simulink model "BuckyWagon_01"  (Simulink 7.7)
settings: Solver=FixedStepDiscrete  StartTime=0.0  StopTime=10.0  RelTol=1e-3
PreLoadFcn:
  | try, eval([bdroot '_setup']); catch, eval('model_setup', ''); end
InitFcn:
  | try, eval([bdroot '_setup']); catch, eval('model_setup', ''); end
undefined symbols (not defined in the file or in its folder): ECU565, High, Low, miniviewSetup, motohawk_build_version, motohawk_get_faults, motohawk_setup_toolchains, motohawk_trunc_name, motohawk_vardec_config_group, motohawk_vardec_path, tc, True
libraries: MotoHawk_lib x594, simulink x27, motohawk_control_primitives_lib x19, miniview_lib x10, MotoHawk_VDOGauge_lib x8, motohawk_engine_lib x5, motohawk_annotations_lib x1
(part 8 of 10)

== system BuckyWagon_01/Foreground/Control Strategy/Drive/HillHold Algorithm ==
  Accel : Inport
  Brake : Inport  Port=2
  Motor_Speed : Inport  Port=3
  Chart : Stateflow chart  TreatAsAtomicUnit=on
  HillHold PI Controller1 : Subsystem
  motohawk_calibration1 : MotoHawk_lib/Calibration & Probing Blocks/motohawk_calibration  nam='HillHoldDisengageBrakePct'  val=0.4  storage=Calibration  show_more=on  name_source=Use Parameter  data_type=Inherit from 'Default Value'  read_level=1  write_level=1  ovr_cals=on  view_as=Number  enum_struct={'Disabled', 'Enabled'}  vector_style=Wide Row  use_help_units=off  help=''  units=''  use_header_enum=off  row_header_enum={}  col_header_enum={}  use_min_max=off  min_val=-inf  max_val=inf  use_precision=off  precision=''  gain=1  offset=0  exp=1  use_mototune_group=off  mototune_group=motohawk_vardec_path(gcb)
  motohawk_calibration2 : MotoHawk_lib/Calibration & Probing Blocks/motohawk_calibration  nam='MinBrakeBedPosforHillHold'  val=0.001  storage=Calibration  show_more=on  name_source=Use Parameter  data_type=Inherit from 'Default Value'  read_level=1  write_level=1  ovr_cals=on  view_as=Number  enum_struct={'Disabled', 'Enabled'}  vector_style=Wide Row  use_help_units=off  help=''  units=''  use_header_enum=off  row_header_enum={}  col_header_enum={}  use_min_max=off  min_val=-inf  max_val=inf  use_precision=off  precision=''  gain=1  offset=0  exp=1  use_mototune_group=off  mototune_group=motohawk_vardec_path(gcb)
  motohawk_probe : MotoHawk_lib/Calibration & Probing Blocks/motohawk_probe  nam='Hill_Hold_On'  show_more=off  name_source=Use Parameter  read_level=1  view_as=Number  enum_struct={'Disabled', 'Enabled'}  vector_style=Wide Row  use_help_units=off  help=''  units=''  use_header_enum=off  row_header_enum={}  col_header_enum={}  use_precision=off  precision=''  gain=1  offset=0  exp=1  use_mototune_group=off  mototune_group=motohawk_vardec_path(gcb)
  HillHoldActive : Outport
  HillHoldTq : Outport  Port=2
  wires:
  Accel/1 -> Chart/1(Accel)
  Brake/1 -> Chart/2(Brake)
  Motor_Speed/1 -> Chart/3(RPM), HillHold PI Controller1/2(RPM)
  motohawk_calibration2/1 -> Chart/4(MinBrakeBedPosforHillHold)
  Chart/1(HillHoldOn) -> HillHoldActive/1, HillHold PI Controller1/1(HillHoldEnable), motohawk_probe/1
  motohawk_calibration1/1 -> Chart/5(HillHoldDisengageBrakePct)
  HillHold PI Controller1/1(HillHoldTq) -> HillHoldTq/1

== system BuckyWagon_01/Foreground/Control Strategy/Drive/Normal Driving ==
  note: This currently does nothing... .005 = 1 clock cycle
  Accel : Inport
  Brake : Inport  Port=2
  SOC : Inport  Port=3
  RPM : Inport  Port=4
  RegenDisabled : Inport  Port=5
  Vehicle Speed : Inport  Port=6
  First Order Low Pass (Tunable) : Subsystem  mask(First-Order Low-Pass Filter (Tunable)){nam='Veh_Speed_Regen_Filter', samp_time=-1, group=motohawk_vardec_path(gcb)}
      mask prompts: nam "Name"; samp_time "Sample Time"; group "MotoTune Group String"
      mask help:
      | Discrete first-order low-pass filter, with calibratable time-constant.
      |
      | If 'Sample Time' is -1, then extra code and RAM will be generated to dynamically calculate dt.
      mask Display:
      | patch([0 0 1 1], [0 0.075 0.075 0], [230/255 0/255 0/255])
      | patch([0 0 1 1], [0.025 0.05 0.05 0.025], [150/255 0/255 0/255])
      | patch([0 0 1 1], [0 0.025 0.025 0], [0/255 0/255 0/255])
      | 
      | disp('1st-Order\nLow Pass');
  First Order Low Pass (Tunable)1 : Subsystem  mask(First-Order Low-Pass Filter (Tunable)){nam='FiltConst', samp_time=-1, group=motohawk_vardec_path(gcb)}
      mask prompts: nam "Name"; samp_time "Sample Time"; group "MotoTune Group String"
      mask help:
      | Discrete first-order low-pass filter, with calibratable time-constant.
      |
      | If 'Sample Time' is -1, then extra code and RAM will be generated to dynamically calculate dt.
      mask Display:
      | patch([0 0 1 1], [0 0.075 0.075 0], [230/255 0/255 0/255])
      | patch([0 0 1 1], [0.025 0.05 0.05 0.025], [150/255 0/255 0/255])
      | patch([0 0 1 1], [0 0.025 0.025 0], [0/255 0/255 0/255])
      | 
      | disp('1st-Order\nLow Pass');
  Logic : Logic  Operator=NOT  AllPortsSameDT=off  OutDataTypeStr=boolean
  Product1 : Product  RndMeth=Zero
  Regen : Subsystem  TreatAsAtomicUnit=on
  Relational Operator2 : RelationalOperator  Operator=>  OutDataTypeStr=boolean
  Switch : Switch  Criteria=u2 ~= 0
  motohawk_calibration1 : MotoHawk_lib/Calibration & Probing Blocks/motohawk_calibration  nam='Max_Slect_Tq_drive'  val=800  storage=Calibration  show_more=off  name_source=Use Parameter  data_type=Inherit from 'Default Value'  read_level=1  write_level=1  ovr_cals=on  view_as=Number  enum_struct={'Disabled', 'Enabled'}  vector_style=Wide Row  use_help_units=off  help=''  units=''  use_header_enum=off  row_header_enum={}  col_header_enum={}  use_min_max=off  min_val=-inf  max_val=inf  use_precision=off  precision=''  gain=1  offset=0  exp=1  use_mototune_group=off  mototune_group=motohawk_vardec_path(gcb)
  motohawk_calibration2 : MotoHawk_lib/Calibration & Probing Blocks/motohawk_calibration  nam='Temp_ped_switchOver'  val=0.005  storage=Calibration  show_more=on  name_source=Use Parameter  data_type=Inherit from 'Default Value'  read_level=1  write_level=1  ovr_cals=on  view_as=Number  enum_struct={'Disabled', 'Enabled'}  vector_style=Wide Row  use_help_units=off  help=''  units=''  use_header_enum=off  row_header_enum={}  col_header_enum={}  use_min_max=off  min_val=-inf  max_val=inf  use_precision=on  precision='1.3'  gain=1  offset=0  exp=1  use_mototune_group=off  mototune_group=motohawk_vardec_path(gcb)
  motohawk_table_1d : MotoHawk_lib/Lookup Tables/motohawk_table_1d  SystemSampleTime=-1  nam='AccelPedalMap'  bp_nam=''  breakpoint_data=[0:.01:1]  table_data="[0\t0\t0\t0.015\t0.03\t0.045\t0.06\t0.075\t0.09\t0.105\t0.12\t0.135\t0.15\t0.165\t0.18\t0.195\t0.21\t0.225\t0.24\t0.255\t0.27\t0.285\t0.3\t0.315\t0.33\t0.345\t0.36\t0.375\t0.39\t0.405\t0.42\t0.435\t0.45\t0.465\t0.48\t0.495\t0.51\t0.525\t0.54\t0.555\t0.57\t0.585\t0.6\t0.615\t0.63\t0.645\t0.66\t0.675\t0.69\t0.7\t0.707106781\t0.714142843\t0.721110255\t0.728010989\t0.734846923\t0.741619849\t0.748331477\t0.754983444\t0.761577311\t0.768114575\t0.774596669\t0.781024968\t0.787400787\t0.793725393\t0.8\t0.806225775\t0.81240384\t0.818535277\t0.824621125\t0.830662386\t0.836660027\t0.842614977\t0.848528137\t0.854400375\t0.860232527\t0.866025404\t0.871779789\t0.877496439\t0.883176087\t0.888819442\t0.894427191\t0.9\t0.905538514\t0.911043358\t0.916515139\t0.921954446\t0.92736185\t0.932737905\t0.938083152\t0.943398113\t0.948683298\t0.953939201\t0.959166305\t0.964365076\t0.969535971\t0.974679434\t0.979795897\t0.98488578\t0.989949494\t0.994987437\t1]"  show_more=on  bp_data_type=Inherit from 'Breakpoint Data'  bp_storage=Constant  table_data_type=Inherit from 'Table Data'  storage=NonAdaptive  read_level=1  write_level=1  ovr_cals=on  use_help=off  help=''  bp_units=''  table_units=''  use_min_max=off  bp_min_val=-inf  bp_max_val=inf  min_val=-inf  max_val=inf  use_precision=on  use_breakpoint=off  b_precision=''  b_gain=1  b_offset=0  b_exp=1  use_table=on  t_precision='1.4'  t_gain=1  t_offset=0  t_exp=1  use_links=off  input_name=''  output_name=''  use_mototune_group=off  mototune_group=motohawk_vardec_path(gcb)
  TorqueReq : Outport
  RegenDisable : Outport  Port=2
  wires:
  First Order Low Pass (Tunable)/1(out) -> Regen/4(RPM)
  Brake/1 -> Regen/2(Brake_Pos)
  motohawk_calibration1/1 -> Product1/1
  Accel/1 -> motohawk_table_1d/1, Relational Operator2/1
  Switch/1 -> TorqueReq/1  "Morot_Torque"
  SOC/1 -> Regen/3(SOC)
  RPM/1 -> First Order Low Pass (Tunable)/1(in)
  RegenDisabled/1 -> Regen/5(RegenDisabled)
  Regen/2(RegenDisable) -> RegenDisable/1  "RegenDisable"
  Product1/1 -> Switch/1
  motohawk_calibration2/1 -> Relational Operator2/2
  Vehicle Speed/1 -> Regen/6(Vehicle Speed)
  Relational Operator2/1 -> Switch/2, Logic/1
  Regen/1(RegenTq) -> First Order Low Pass (Tunable)1/1(in)
  Logic/1 -> Regen/1(switch active)
  First Order Low Pass (Tunable)1/1(out) -> Switch/3
  motohawk_table_1d/1 -> Product1/2

== system BuckyWagon_01/Foreground/Control Strategy/HV Controller/Contacter Controller ==
  Battery OK : Inport  OutDataTypeStr=boolean
  Shutdown Command : Inport  Port=2  OutDataTypeStr=boolean
  Contactor Status : Inport  Port=3  OutDataTypeStr=boolean
  Delay falling edge : Subsystem
  Delay rising edge : Subsystem
  Logical Operator2 : Logic  AllPortsSameDT=off  OutDataTypeStr=boolean
  Logical Operator3 : Logic  Operator=NOT  AllPortsSameDT=off  OutDataTypeStr=boolean
  Logical Operator4 : Logic  Inputs=3  AllPortsSameDT=off  OutDataTypeStr=boolean
  Logical Operator5 : Logic  Operator=NOT  AllPortsSameDT=off  OutDataTypeStr=boolean
  Logical Operator6 : Logic  Operator=NOT  AllPortsSameDT=off  OutDataTypeStr=boolean
  Relational Operator : RelationalOperator  OutDataTypeStr=boolean
  Relational Operator1 : RelationalOperator  OutDataTypeStr=boolean
  Time Since Enabled (With Input)1 : motohawk_control_primitives_lib/Time Since Enabled (With Input)1  SystemSampleTime=-1  nam='Contactor_Disable_Timer'  samp_time=-1  init=0  upperlim=3600*24
  Time Since Enabled (With Input)3 : motohawk_control_primitives_lib/Time Since Enabled (With Input)1  SystemSampleTime=-1  nam='Solectria_Enable_timer'  samp_time=-1  init=0  upperlim=3600*24
  motohawk_calibration : MotoHawk_lib/Calibration & Probing Blocks/motohawk_calibration  nam='Contactor_Disable_Delay'  val=0.5  storage=Calibration  show_more=on  name_source=Use Parameter  data_type=Inherit from 'Default Value'  read_level=1  write_level=1  ovr_cals=on  view_as=Number  enum_struct={'Disabled', 'Enabled'}  vector_style=Wide Row  use_help_units=off  help=''  units=''  use_header_enum=off  row_header_enum={}  col_header_enum={}  use_min_max=on  min_val=0  max_val=10  use_precision=on  precision='1.2'  gain=1  offset=0  exp=1  use_mototune_group=on  mototune_group=motohawk_vardec_path(gcb)
  motohawk_calibration1 : MotoHawk_lib/Calibration & Probing Blocks/motohawk_calibration  nam='Load_Enable_Delay'  val=2  storage=Calibration  show_more=on  name_source=Use Parameter  data_type=Inherit from 'Default Value'  read_level=1  write_level=1  ovr_cals=on  view_as=Number  enum_struct={'Disabled', 'Enabled'}  vector_style=Wide Row  use_help_units=off  help=''  units=''  use_header_enum=off  row_header_enum={}  col_header_enum={}  use_min_max=on  min_val=0  max_val=10  use_precision=on  precision='1.2'  gain=1  offset=0  exp=1  use_mototune_group=on  mototune_group=motohawk_vardec_path(gcb)
  motohawk_data_write : MotoHawk_lib/Data Storage Blocks/motohawk_data_write  source=Lookup By Name  structure=Scalar  operation=Write entire data structure at once  sz_vec=-1  sz_row=3  sz_col=2  typ=boolean  nam='MPRD_KeepAlive'  checkNull=off  write_read_only=off  struct_inst_name='Struct1'  struct_name='MyStruct'
  Contactor Enable : Outport  OutDataTypeStr=boolean
  Load Enable : Outport  Port=2  OutDataTypeStr=boolean
  wires:
  Time Since Enabled (With Input)1/1 -> Relational Operator/1
  Logical Operator3/1 -> Logical Operator4/1
  Time Since Enabled (With Input)3/1 -> Relational Operator1/1
  Relational Operator1/1 -> Logical Operator4/2
  Logical Operator5/1 -> Time Since Enabled (With Input)3/1
  Logical Operator4/1 -> Load Enable/1
  motohawk_calibration/1 -> Relational Operator/2
  motohawk_calibration1/1 -> Relational Operator1/2
  Relational Operator/1 -> Logical Operator6/1
  Logical Operator6/1 -> Logical Operator2/2
  Battery OK/1 -> Delay rising edge/1(In)
  Delay falling edge/1(Out) -> motohawk_data_write/1
  Contactor Status/1 -> Logical Operator4/3
  Delay rising edge/1(Out) -> Logical Operator2/1
  Logical Operator2/1 -> Contactor Enable/1, Delay falling edge/1(In)
  Shutdown Command/1 -> Time Since Enabled (With Input)1/1, Logical Operator5/1, Logical Operator3/1

== system BuckyWagon_01/Foreground/MiniViewDisplay/Down Button/Subsystem ==
  Trigger : TriggerPort  TriggerType=function-call
  Read CAN Message : MotoHawk_lib/CAN Blocks/Read CAN Message  nam=['CAN_' num2str(miniview_CAN_channel)]  bus=-2  msg=miniview_button_down  queue=1  slot='miniview_button_down'  valid=off  stale=off  labelwires=on
  Signal Specification : SignalSpecification  OutDataTypeStr=boolean
  Signal Specification1 : SignalSpecification  OutDataTypeStr=uint8
  Out1 : Outport
  Out2 : Outport  Port=2
  wires:
  Signal Specification1/1 -> Out2/1  "down count"
  Signal Specification/1 -> Out1/1  "down asserted"
  Read CAN Message/2 -> Signal Specification1/1  "down count"
  Read CAN Message/1 -> Signal Specification/1  "down asserted"

== system BuckyWagon_01/Foreground/MiniViewDisplay/GetFaultName/Fault Iterator ==
  function : TriggerPort  TriggerType=function-call
  Unit Delay : UnitDelay  SampleTime=-1
  motohawk_fault_iterator : MotoHawk_lib/Fault Management Blocks/motohawk_fault_iterator  criteria=Active Faults  loop=on
  motohawk_fault_name : MotoHawk_lib/Fault Management Blocks/motohawk_fault_name  width=size(char(motohawk_get_faults),2)+1
  Name : Outport
  valid : Outport  Port=2
  wires:
  motohawk_fault_iterator/2 -> Unit Delay/1, motohawk_fault_name/1
  Unit Delay/1 -> motohawk_fault_iterator/1
  motohawk_fault_iterator/1 -> valid/1
  motohawk_fault_name/1 -> Name/1

== system BuckyWagon_01/Foreground/MiniViewDisplay/Menu Button/Subsystem ==
  Trigger : TriggerPort  TriggerType=function-call
  Read CAN Message : MotoHawk_lib/CAN Blocks/Read CAN Message  nam=['CAN_' num2str(miniview_CAN_channel)]  bus=-2  msg=miniview_button_menu  queue=1  slot='miniview_button_menu'  valid=off  stale=off  labelwires=on
  Signal Specification : SignalSpecification  OutDataTypeStr=boolean
  Signal Specification1 : SignalSpecification  OutDataTypeStr=uint8
  Out1 : Outport
  Out2 : Outport  Port=2
  wires:
  Read CAN Message/1 -> Signal Specification/1  "menu asserted"
  Read CAN Message/2 -> Signal Specification1/1  "menu count"
  Signal Specification/1 -> Out1/1  "menu asserted"
  Signal Specification1/1 -> Out2/1  "menu count"

== system BuckyWagon_01/Foreground/MiniViewDisplay/Send String_efficient/Subsystem ==
  string # : Inport
  string : Inport  Port=2
  Trigger : TriggerPort  TriggerType=function-call
  Demux3 : Demux  Outputs=[7 7 3 1]
  Function-Call Generator : simulink/Ports & Subsystems/Function-Call Generator  sample_time=-1  numberOfIterations=1
  Function-Call Subsystem : Subsystem  TreatAsAtomicUnit=on
  Function-Call Subsystem1 : Subsystem  TreatAsAtomicUnit=on
  Send Substring (page 0) : miniview_lib/Send Substring (page 0)  SystemSampleTime=-1  miniview_CAN_channel=miniview_CAN_channel
  Send Substring (page 1) : miniview_lib/Send Substring (page 1)  SystemSampleTime=-1  miniview_CAN_channel=miniview_CAN_channel
  Send Substring (page 2) : miniview_lib/Send Substring (page 2)  SystemSampleTime=-1  miniview_CAN_channel=miniview_CAN_channel
  Terminator : Terminator
  Terminator1 : Terminator
  wires:
  Demux3/3 -> Send Substring (page 2)/2
  Demux3/2 -> Send Substring (page 1)/2, Function-Call Subsystem1/1(In1)
  Demux3/1 -> Send Substring (page 0)/2, Function-Call Subsystem/1(In1)
  string/1 -> Demux3/1  "string"
  string #/1 -> Send Substring (page 1)/1, Send Substring (page 2)/1, Send Substring (page 0)/1  "string #"
  Function-Call Generator/1 -> Send Substring (page 0)/Trigger
  Send Substring (page 0)/1 -> Function-Call Subsystem/Trigger
  Function-Call Subsystem/1(Out) -> Send Substring (page 1)/Trigger
  Send Substring (page 1)/1 -> Function-Call Subsystem1/Trigger
  Function-Call Subsystem1/1(Out) -> Send Substring (page 2)/Trigger
  Demux3/4 -> Terminator/1
  Send Substring (page 2)/1 -> Terminator1/1

== system BuckyWagon_01/Foreground/MiniViewDisplay/Up Button/Subsystem ==
  Trigger : TriggerPort  TriggerType=function-call
  Read CAN Message : MotoHawk_lib/CAN Blocks/Read CAN Message  nam=['CAN_' num2str(miniview_CAN_channel)]  bus=-2  msg=miniview_button_up  queue=1  slot='miniview_button_up'  valid=off  stale=off  labelwires=on
  Signal Specification : SignalSpecification  OutDataTypeStr=boolean
  Signal Specification1 : SignalSpecification  OutDataTypeStr=uint8
  Up Asserted : Outport
  Up Count : Outport  Port=2
  wires:
  Signal Specification1/1 -> Up Count/1  "up count"
  Signal Specification/1 -> Up Asserted/1  "up asserted"
  Read CAN Message/2 -> Signal Specification1/1  "up count"
  Read CAN Message/1 -> Signal Specification/1  "up asserted"

== system BuckyWagon_01/Foreground/Sensors/Brusa Charger/PluggedInDetect ==
  MainsVolt : Inport
  Thres : Inport  Port=2
  Time : Inport  Port=3
  Chart : Stateflow chart  TreatAsAtomicUnit=on
  Relational Operator : RelationalOperator  Operator=>  OutDataTypeStr=boolean
  pluggedIn : Outport
  wires:
  MainsVolt/1 -> Relational Operator/1
  Thres/1 -> Relational Operator/2
  Chart/1(pluggedIn) -> pluggedIn/1
  Relational Operator/1 -> Chart/2(mainsOn)
  Time/1 -> Chart/1(histTime)

== system BuckyWagon_01/Foreground/Sensors/Eaton HV Charger/PluggedInDetect ==
  MainsVolt : Inport
  Thres : Inport  Port=2
  Time : Inport  Port=3
  Chart : Stateflow chart  TreatAsAtomicUnit=on
  Relational Operator : RelationalOperator  Operator=>  OutDataTypeStr=boolean
  pluggedIn : Outport
  wires:
  MainsVolt/1 -> Relational Operator/1
  Thres/1 -> Relational Operator/2
  Chart/1(pluggedIn) -> pluggedIn/1
  Relational Operator/1 -> Chart/2(mainsOn)
  Time/1 -> Chart/1(histTime)

== system BuckyWagon_01/Foreground/Sensors/Linear Sensor Characterization/If Action Subsystem ==
  In : Inport
  Action Port : ActionPort  ActionType=then
  Out : Outport
  wires:
  In/1 -> Out/1

== system BuckyWagon_01/Foreground/Sensors/Linear Sensor Characterization/If Action Subsystem1 ==
  In : Inport
  Action Port : ActionPort  ActionType=elseif
  Out : Outport
  wires:
  In/1 -> Out/1

== system BuckyWagon_01/Foreground/Sensors/Linear Sensor Characterization/If Action Subsystem2 ==
  In : Inport
  Action Port : ActionPort  ActionType=else
  Out : Outport
  wires:
  In/1 -> Out/1

== system BuckyWagon_01/Foreground/Sensors/Linear Sensor Characterization2/If Action Subsystem ==
  In : Inport
  Action Port : ActionPort  ActionType=then
  Out : Outport
  wires:
  In/1 -> Out/1

== system BuckyWagon_01/Foreground/Sensors/Linear Sensor Characterization2/If Action Subsystem1 ==
  In : Inport
  Action Port : ActionPort  ActionType=elseif
  Out : Outport
  wires:
  In/1 -> Out/1

== system BuckyWagon_01/Foreground/Sensors/Linear Sensor Characterization2/If Action Subsystem2 ==
  In : Inport
  Action Port : ActionPort  ActionType=else
  Out : Outport
  wires:
  In/1 -> Out/1

== system BuckyWagon_01/Main Power Relay/Background/Delay/MotoHawk S-R Flip-Flop ==
  note: MotoHawk S-R Flip-Flop
  S : Inport
  R : Inport  Port=2
  Logical Operator : Logic  Operator=OR  OutDataTypeStr=boolean
  Logical Operator1 : Logic  Operator=NOT  OutDataTypeStr=boolean
  Logical Operator2 : Logic  OutDataTypeStr=boolean
  Logical Operator3 : Logic  Operator=NOT  OutDataTypeStr=boolean
  Signal Specification : SignalSpecification  OutDataTypeStr=boolean
  Signal Specification1 : SignalSpecification  OutDataTypeStr=boolean
  Unit Delay : UnitDelay  X0=ic_bool  SampleTime=-1
  Q : Outport
  !Q : Outport  Port=2
  wires:
  Logical Operator3/1 -> !Q/1
  R/1 -> Signal Specification/1
  S/1 -> Signal Specification1/1
  Signal Specification1/1 -> Logical Operator/2
  Signal Specification/1 -> Logical Operator1/1
  Logical Operator2/1 -> Q/1, Unit Delay/1, Logical Operator3/1
  Unit Delay/1 -> Logical Operator/1
  Logical Operator/1 -> Logical Operator2/1
  Logical Operator1/1 -> Logical Operator2/2

== system BuckyWagon_01/Foreground/Actuators/Analog Out/ReverseInd/Enabled Subsystem ==
  Period (Cnt) : Inport
  Enable : EnablePort  StatesWhenEnabling=reset
  Constant : Constant  OutDataTypeStr=int16
  Gain : Gain  Gain=0.5  OutDataTypeStr=Inherit: Same as input
  Relational Operator : RelationalOperator  Operator=<=  OutDataTypeStr=boolean
  Sum : Sum  Inputs=|+-
  Switch : Switch  Criteria=u2 > Threshold
  Unit Delay : UnitDelay  SampleTime=-1
  Out : Outport  InitialOutput=[0]
  wires:
  Relational Operator/1 -> Out/1
  Gain/1 -> Relational Operator/1
  Period (Cnt)/1 -> Gain/1, Switch/3
  Switch/1 -> Sum/1
  Sum/1 -> Relational Operator/2, Unit Delay/1
  Unit Delay/1 -> Switch/1, Switch/2
  Constant/1 -> Sum/2

== system BuckyWagon_01/Foreground/Addl_Fault_Detection/Battery/Over_Under_SOC_Management/SOCAlert ==
  note: 78%=399.8V
  CurrentSOC : Inport
  Relational Operator : RelationalOperator  Operator=<=  OutDataTypeStr=boolean
  Relational Operator1 : RelationalOperator  Operator=<=  OutDataTypeStr=boolean
  motohawk_calibration1 : MotoHawk_lib/Calibration & Probing Blocks/motohawk_calibration  nam='Under_SOCAlertThresh'  val=26  storage=Calibration  show_more=on  name_source=Use Parameter  data_type=Inherit from 'Default Value'  read_level=1  write_level=1  ovr_cals=on  view_as=Number  enum_struct={'Disabled', 'Enabled'}  vector_style=Wide Row  use_help_units=on  help=''  units='Percent above or below the JCS specified limits that a warning will be issued'  use_header_enum=off  row_header_enum={}  col_header_enum={}  use_min_max=off  min_val=-inf  max_val=inf  use_precision=off  precision=''  gain=1  offset=0  exp=1  use_mototune_group=off  mototune_group=motohawk_vardec_path(gcb)
  motohawk_calibration2 : MotoHawk_lib/Calibration & Probing Blocks/motohawk_calibration  nam='Over_SOCAlertThresh'  val=100  storage=Calibration  show_more=on  name_source=Use Parameter  data_type=Inherit from 'Default Value'  read_level=1  write_level=1  ovr_cals=on  view_as=Number  enum_struct={'Disabled', 'Enabled'}  vector_style=Wide Row  use_help_units=on  help=''  units=''  use_header_enum=off  row_header_enum={}  col_header_enum={}  use_min_max=off  min_val=-inf  max_val=inf  use_precision=off  precision=''  gain=1  offset=0  exp=1  use_mototune_group=off  mototune_group=motohawk_vardec_path(gcb)
  OverSOCAlert : Outport
  UnderSOCAlert : Outport  Port=2
  wires:
  CurrentSOC/1 -> Relational Operator/2, Relational Operator1/1
  motohawk_calibration1/1 -> Relational Operator1/2
  Relational Operator/1 -> OverSOCAlert/1
  Relational Operator1/1 -> UnderSOCAlert/1
  motohawk_calibration2/1 -> Relational Operator/1

== system BuckyWagon_01/Foreground/Addl_Fault_Detection/Battery/Over_Under_SOC_Management/SOCShutdown ==
  CurrentSOC : Inport
  Relational Operator : RelationalOperator  Operator=<=  OutDataTypeStr=boolean
  Relational Operator1 : RelationalOperator  Operator=<=  OutDataTypeStr=boolean
  motohawk_calibration1 : MotoHawk_lib/Calibration & Probing Blocks/motohawk_calibration  nam='Under_SOC_Shutdown_Thresh'  val=21  storage=Calibration  show_more=on  name_source=Use Parameter  data_type=Inherit from 'Default Value'  read_level=1  write_level=1  ovr_cals=on  view_as=Number  enum_struct={'Disabled', 'Enabled'}  vector_style=Wide Row  use_help_units=on  help=''  units=''  use_header_enum=off  row_header_enum={}  col_header_enum={}  use_min_max=off  min_val=-inf  max_val=inf  use_precision=off  precision=''  gain=1  offset=0  exp=1  use_mototune_group=off  mototune_group=motohawk_vardec_path(gcb)
  motohawk_calibration2 : MotoHawk_lib/Calibration & Probing Blocks/motohawk_calibration  nam='Over_SOC_Shutdown_Thresh'  val=101  storage=Calibration  show_more=on  name_source=Use Parameter  data_type=Inherit from 'Default Value'  read_level=1  write_level=1  ovr_cals=on  view_as=Number  enum_struct={'Disabled', 'Enabled'}  vector_style=Wide Row  use_help_units=on  help=''  units=''  use_header_enum=off  row_header_enum={}  col_header_enum={}  use_min_max=off  min_val=-inf  max_val=inf  use_precision=off  precision=''  gain=1  offset=0  exp=1  use_mototune_group=off  mototune_group=motohawk_vardec_path(gcb)
  OverSOCAlert : Outport
  UnderSOCAlert : Outport  Port=2
  wires:
  CurrentSOC/1 -> Relational Operator/2, Relational Operator1/1
  motohawk_calibration1/1 -> Relational Operator1/2
  Relational Operator/1 -> OverSOCAlert/1
  Relational Operator1/1 -> UnderSOCAlert/1
  motohawk_calibration2/1 -> Relational Operator/1

== system BuckyWagon_01/Foreground/Addl_Fault_Detection/Traction Drive/Hysterisis/Hysteresis ==
  note: Hi & !Lo => Hi
      | Lo & !Hi => Lo
      | Otherwise, Hold
  Hi : Inport
  Lo : Inport  Port=2
  Combinatorial  Logic : CombinatorialLogic  TruthTable=[0 0;0 1;1 1;0 0]
  Demux : Demux  Outputs=2
  Mux : Mux  Inputs=2
  Switch1 : Switch  Threshold=0.5  SaturateOnIntegerOverflow=on  InputSameDT=on
  Unit Delay : UnitDelay  SampleTime=-1
  "Out (Lo=0, Hi=1)" : Outport
  wires:
  Mux/1 -> Combinatorial  Logic/1
  Combinatorial  Logic/1 -> Demux/1
  Demux/1 -> Switch1/1
  Demux/2 -> Switch1/2
  Unit Delay/1 -> Switch1/3
  Switch1/1 -> Unit Delay/1, "Out (Lo=0, Hi=1)"/1
  Hi/1 -> Mux/1
  Lo/1 -> Mux/2

== system BuckyWagon_01/Foreground/Control Strategy/Drive/HillHold Algorithm/HillHold PI Controller1 ==
  HillHoldEnable : Inport
  RPM : Inport  Port=2
  Constant : Constant  Value=0
  First Order Low Pass (Tunable) : Subsystem  mask(First-Order Low-Pass Filter (Tunable)){nam='UQM_HillHoldSpeed_Filt', samp_time=-1, group=motohawk_vardec_path(gcb)}
      mask prompts: nam "Name"; samp_time "Sample Time"; group "MotoTune Group String"
      mask help:
      | Discrete first-order low-pass filter, with calibratable time-constant.
      |
      | If 'Sample Time' is -1, then extra code and RAM will be generated to dynamically calculate dt.
      mask Display:
      | patch([0 0 1 1], [0 0.075 0.075 0], [230/255 0/255 0/255])
      | patch([0 0 1 1], [0.025 0.05 0.05 0.025], [150/255 0/255 0/255])
      | patch([0 0 1 1], [0 0.025 0.025 0], [0/255 0/255 0/255])
      | 
      | disp('1st-Order\nLow Pass');
  Product : Product  RndMeth=Zero
  Rising Edge : motohawk_control_primitives_lib/Rising Edge  SystemSampleTime=-1
  Saturation1 : motohawk_control_primitives_lib/Saturation  SystemSampleTime=-1
  Simple PI : Subsystem  Description=|  AncestorBlock=motohawk_control_primitives_lib/Simple PI  mask(Universal PID){samp_time=-1}
      | /* Name: ErrorGain Unit:mult ClassID:VAR StorageID:FLASH Access:RW4+RW3+NA2+NA1 TypeID:UINT4                   
      |    Gain:0.000000001 Min:0.000000000 Max:4.000000000 Format:10.9 UpdateID:REMOTE Help:"This gain is applied to "
      |    "the error term before it is used to calculate the P, I and D terms." VardecSig:6C */                       
      |                                                                                                                
      | /* Name: ITermLowerLim Unit:0 ClassID:VAR StorageID:FLASH Access:RW4+RW3+NA2+NA1 TypeID:SINT2 Gain:0.1         
      |    Min:-3276.8 Max:3276.7 Format:5.1 UpdateID:REMOTE Help:"Lower limit on the I-term value." VardecSig:6C */   
      |                                                                                                                
      | /* Name: ITermUpperLim ClassID:VAR StorageID:FLASH Access:RW4+RW3+NA2+NA1 TypeID:SINT2 Gain:0.1 Min:-3276.8    
      |    Max:3276.7 Format:5.1 UpdateID:REMOTE Help:"Upper limit on I-term value." VardecSig:6C */                   
      |                                                                                                                
      | /* Name: PIDOutLowerLim ClassID:VAR StorageID:FLASH Access:RW4+RW3+NA2+NA1 TypeID:SINT2 Gain:0.1               
      |    Min:-3276.8 Max:3276.7 Format:5.1 UpdateID:REMOTE Help:"Lower limit on PID output." VardecSig:6C */         
      |                                                                                                                
      | /* Name: PIDOutUpperLim ClassID:VAR StorageID:FLASH Access:RW4+RW3+NA2+NA1 TypeID:SINT2 Gain:0.1               
      |    Min:-3276.8 Max:3276.7 Format:3.1 UpdateID:REMOTE Help:"Upper limit on PID output." VardecSig:6C */
      mask prompts: samp_time "Sample Time"
      mask help:
      | Resettable PID controller with limits on the I-term.
      |
      | If 'Sample Time' is -1, then extra code and RAM will be generated to dynamically calculate dt.
      mask Display:
      | patch([0 0 1 1], 0.75*[0 0.075 0.075 0], [230/255 0/255 0/255])
      | patch([0 0 1 1], 0.75*[0.025 0.05 0.05 0.025], [150/255 0/255 0/255])
      | patch([0 0 1 1], 0.75*[0 0.025 0.025 0], [0/255 0/255 0/255])
      | 
      | disp('\fontsize{16}\bf\itPI', 'texmode', 'on');
  motohawk_calibration1 : MotoHawk_lib/Calibration & Probing Blocks/motohawk_calibration  nam='HillHold_kP'  val=0.4  storage=Calibration  show_more=on  name_source=Use Parameter  data_type=Inherit from 'Default Value'  read_level=1  write_level=1  ovr_cals=on  view_as=Number  enum_struct={'Disabled', 'Enabled'}  vector_style=Wide Row  use_help_units=off  help=''  units=''  use_header_enum=off  row_header_enum={}  col_header_enum={}  use_min_max=off  min_val=-inf  max_val=inf  use_precision=off  precision=''  gain=1  offset=0  exp=1  use_mototune_group=off  mototune_group=motohawk_vardec_path(gcb)
  motohawk_calibration2 : MotoHawk_lib/Calibration & Probing Blocks/motohawk_calibration  nam='HillHoldMaxREVTqSaturation'  val=0  storage=Calibration  show_more=on  name_source=Use Parameter  data_type=Inherit from 'Default Value'  read_level=1  write_level=1  ovr_cals=on  view_as=Number  enum_struct={'Disabled', 'Enabled'}  vector_style=Wide Row  use_help_units=off  help=''  units=''  use_header_enum=off  row_header_enum={}  col_header_enum={}  use_min_max=off  min_val=-inf  max_val=inf  use_precision=off  precision=''  gain=1  offset=0  exp=1  use_mototune_group=off  mototune_group=motohawk_vardec_path(gcb)
  motohawk_calibration3 : MotoHawk_lib/Calibration & Probing Blocks/motohawk_calibration  nam='HillHold_kI'  val=.6  storage=Calibration  show_more=on  name_source=Use Parameter  data_type=Inherit from 'Default Value'  read_level=1  write_level=1  ovr_cals=on  view_as=Number  enum_struct={'Disabled', 'Enabled'}  vector_style=Wide Row  use_help_units=off  help=''  units=''  use_header_enum=off  row_header_enum={}  col_header_enum={}  use_min_max=off  min_val=-inf  max_val=inf  use_precision=off  precision=''  gain=1  offset=0  exp=1  use_mototune_group=off  mototune_group=motohawk_vardec_path(gcb)
  motohawk_calibration4 : MotoHawk_lib/Calibration & Probing Blocks/motohawk_calibration  nam='HillHoldTorqueGain'  val=1.45  storage=Calibration  show_more=on  name_source=Use Parameter  data_type=Inherit from 'Default Value'  read_level=1  write_level=1  ovr_cals=on  view_as=Number  enum_struct={'Disabled', 'Enabled'}  vector_style=Wide Row  use_help_units=off  help=''  units=''  use_header_enum=off  row_header_enum={}  col_header_enum={}  use_min_max=off  min_val=-inf  max_val=inf  use_precision=off  precision=''  gain=1  offset=0  exp=1  use_mototune_group=off  mototune_group=motohawk_vardec_path(gcb)
  motohawk_calibration5 : MotoHawk_lib/Calibration & Probing Blocks/motohawk_calibration  nam='HillHoldMaxFWDTqSaturation'  val=70  storage=Calibration  show_more=on  name_source=Use Parameter  data_type=Inherit from 'Default Value'  read_level=1  write_level=1  ovr_cals=on  view_as=Number  enum_struct={'Disabled', 'Enabled'}  vector_style=Wide Row  use_help_units=off  help=''  units=''  use_header_enum=off  row_header_enum={}  col_header_enum={}  use_min_max=off  min_val=-inf  max_val=inf  use_precision=off  precision=''  gain=1  offset=0  exp=1  use_mototune_group=off  mototune_group=motohawk_vardec_path(gcb)
  motohawk_probe1 : MotoHawk_lib/Calibration & Probing Blocks/motohawk_probe  nam='HillHoldPI_Output'  show_more=off  name_source=Use Parameter  read_level=1  view_as=Number  enum_struct={'Disabled', 'Enabled'}  vector_style=Wide Row  use_help_units=off  help=''  units=''  use_header_enum=off  row_header_enum={}  col_header_enum={}  use_precision=off  precision=''  gain=1  offset=0  exp=1  use_mototune_group=off  mototune_group=motohawk_vardec_path(gcb)
  motohawk_probe2 : MotoHawk_lib/Calibration & Probing Blocks/motohawk_probe  nam='HillHold_UQMSpeed_Postfilt'  show_more=off  name_source=Use Parameter  read_level=1  view_as=Number  enum_struct={'Disabled', 'Enabled'}  vector_style=Wide Row  use_help_units=off  help=''  units=''  use_header_enum=off  row_header_enum={}  col_header_enum={}  use_precision=off  precision=''  gain=1  offset=0  exp=1  use_mototune_group=off  mototune_group=motohawk_vardec_path(gcb)
  HillHoldTq : Outport
  wires:
  Saturation1/1 -> HillHoldTq/1
  HillHoldEnable/1 -> Rising Edge/1
  RPM/1 -> First Order Low Pass (Tunable)/1(in)
  motohawk_calibration5/1 -> Saturation1/3
  motohawk_calibration2/1 -> Saturation1/2
  Product/1 -> Saturation1/1
  motohawk_calibration4/1 -> Product/1
  Simple PI/1(Out) -> Product/2, motohawk_probe1/1
  Rising Edge/1 -> Simple PI/5(IC Reset)
  motohawk_calibration3/1 -> Simple PI/4(k_I)
  motohawk_calibration1/1 -> Simple PI/3(k_P)
  Constant/1 -> Simple PI/2(SetPt)
  First Order Low Pass (Tunable)/1(out) -> motohawk_probe2/1, Simple PI/1(Actual)

== system BuckyWagon_01/Foreground/Control Strategy/Drive/Normal Driving/First Order Low Pass (Tunable) ==
  note: Tunable 1st-Order Low-Pass Filter
  in : Inport
  First Order Low Pass : motohawk_control_primitives_lib/First Order Low Pass  SystemSampleTime=-1
  MinMax : MinMax  Function=max  Inputs=2  SaturateOnIntegerOverflow=on  InputSameDT=on
  Product : Product  Inputs=*/  SaturateOnIntegerOverflow=on  InputSameDT=on  OutDataTypeStr=Inherit: Same as first input
  motohawk_calibration : MotoHawk_lib/Calibration & Probing Blocks/motohawk_calibration  nam=nam  val=0.1  storage=Calibration  show_more=on  name_source=Use Parameter  data_type=Inherit from 'Default Value'  read_level=1  write_level=1  ovr_cals=on  view_as=Number  enum_struct={'Disabled', 'Enabled'}  vector_style=Wide Row  use_help_units=on  help='Filter time constant'  units='sec'  use_header_enum=off  row_header_enum={}  col_header_enum={}  use_min_max=off  min_val=-inf  max_val=inf  use_precision=off  precision=''  gain=1  offset=0  exp=1  use_mototune_group=on  mototune_group=group %% motohawk_vardec_config_group(group)
  motohawk_delta_time : MotoHawk_lib/Extra Development Blocks/motohawk_delta_time  samp_time=samp_time  init_val=0  mode=Seconds (double)
  out : Outport
  wires:
  First Order Low Pass/1 -> out/1
  in/1 -> First Order Low Pass/1
  motohawk_delta_time/1 -> Product/1, MinMax/1
  Product/1 -> First Order Low Pass/2
  MinMax/1 -> Product/2
  motohawk_calibration/1 -> MinMax/2

== system BuckyWagon_01/Foreground/Control Strategy/Drive/Normal Driving/First Order Low Pass (Tunable)1 ==
  note: Tunable 1st-Order Low-Pass Filter
  in : Inport
  First Order Low Pass : motohawk_control_primitives_lib/First Order Low Pass  SystemSampleTime=-1
  MinMax : MinMax  Function=max  Inputs=2  SaturateOnIntegerOverflow=on  InputSameDT=on
  Product : Product  Inputs=*/  SaturateOnIntegerOverflow=on  InputSameDT=on  OutDataTypeStr=Inherit: Same as first input
  motohawk_calibration : MotoHawk_lib/Calibration & Probing Blocks/motohawk_calibration  nam='Regin_torque_const'  val=.01  storage=Calibration  show_more=on  name_source=Use Parameter  data_type=Inherit from 'Default Value'  read_level=1  write_level=1  ovr_cals=on  view_as=Number  enum_struct={'Disabled', 'Enabled'}  vector_style=Wide Row  use_help_units=on  help='Filter time constant'  units='sec'  use_header_enum=off  row_header_enum={}  col_header_enum={}  use_min_max=off  min_val=-inf  max_val=inf  use_precision=off  precision=''  gain=1  offset=0  exp=1  use_mototune_group=on  mototune_group=group %% motohawk_vardec_config_group(group)
  motohawk_delta_time : MotoHawk_lib/Extra Development Blocks/motohawk_delta_time  samp_time=samp_time  init_val=0  mode=Seconds (double)
  out : Outport
  wires:
  First Order Low Pass/1 -> out/1
  in/1 -> First Order Low Pass/1
  motohawk_delta_time/1 -> Product/1, MinMax/1
  Product/1 -> First Order Low Pass/2
  MinMax/1 -> Product/2
  motohawk_calibration/1 -> MinMax/2

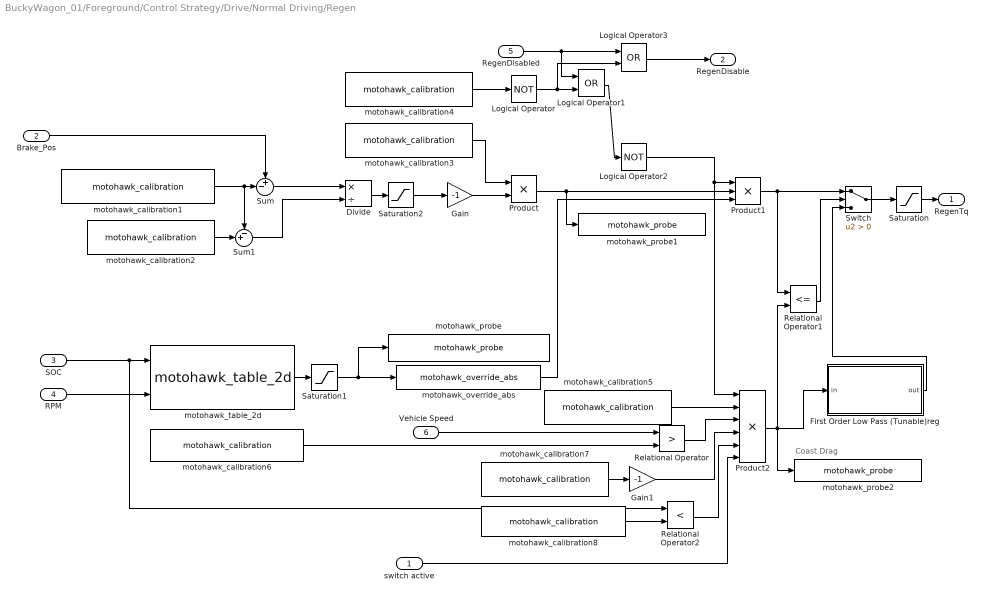
== system BuckyWagon_01/Foreground/Control Strategy/Drive/Normal Driving/Regen ==
  note: Coast Drag
  switch active : Inport
  Brake_Pos : Inport  Port=2
  SOC : Inport  Port=3
  RPM : Inport  Port=4
  RegenDisabled : Inport  Port=5
  Vehicle Speed : Inport  Port=6
  Divide : Product  Inputs=*/
  First Order Low Pass (Tunable)reg : Subsystem  mask(First-Order Low-Pass Filter (Tunable)){nam='FiltConst', samp_time=-1, group=motohawk_vardec_path(gcb)}
      mask prompts: nam "Name"; samp_time "Sample Time"; group "MotoTune Group String"
      mask help:
      | Discrete first-order low-pass filter, with calibratable time-constant.
      |
      | If 'Sample Time' is -1, then extra code and RAM will be generated to dynamically calculate dt.
      mask Display:
      | patch([0 0 1 1], [0 0.075 0.075 0], [230/255 0/255 0/255])
      | patch([0 0 1 1], [0.025 0.05 0.05 0.025], [150/255 0/255 0/255])
      | patch([0 0 1 1], [0 0.025 0.025 0], [0/255 0/255 0/255])
      | 
      | disp('1st-Order\nLow Pass');
  Gain : Gain  Gain=-1
  Gain1 : Gain  Gain=-1
  Logical Operator : Logic  Operator=NOT  AllPortsSameDT=off  OutDataTypeStr=boolean
  Logical Operator1 : Logic  Operator=OR  AllPortsSameDT=off  OutDataTypeStr=boolean
  Logical Operator2 : Logic  Operator=NOT  AllPortsSameDT=off  OutDataTypeStr=boolean
  Logical Operator3 : Logic  Operator=OR  AllPortsSameDT=off  OutDataTypeStr=boolean
  Product : Product  RndMeth=Zero
  Product1 : Product  Inputs=3  RndMeth=Zero
  Product2 : Product  Inputs=6  RndMeth=Zero
  Relational Operator : RelationalOperator  Operator=>  OutDataTypeStr=boolean
  Relational Operator1 : RelationalOperator  Operator=<=  OutDataTypeStr=boolean
  Relational Operator2 : RelationalOperator  Operator=<  OutDataTypeStr=boolean
  Saturation : Saturate  UpperLimit=0  LowerLimit=-240
  Saturation1 : Saturate  UpperLimit=1  LowerLimit=0
  Saturation2 : Saturate  UpperLimit=1  LowerLimit=0
  Sum : Sum  Inputs=+-|
  Sum1 : Sum  Inputs=-+|
  Switch : Switch  Criteria=u2 > Threshold
  motohawk_calibration1 : MotoHawk_lib/Calibration & Probing Blocks/motohawk_calibration  nam='Regen_Start'  val=0.03  storage=Calibration  show_more=on  name_source=Use Parameter  data_type=Inherit from 'Default Value'  read_level=1  write_level=1  ovr_cals=on  view_as=Number  enum_struct={'Disabled', 'Enabled'}  vector_style=Wide Row  use_help_units=on  help='AKA deadband, Pedal Position where regen is at min'  units='%'  use_header_enum=off  row_header_enum={}  col_header_enum={}  use_min_max=on  min_val=0  max_val=1  use_precision=off  precision='1.2'  gain=1  offset=0  exp=1  use_mototune_group=off  mototune_group=motohawk_vardec_path(gcb)
  motohawk_calibration2 : MotoHawk_lib/Calibration & Probing Blocks/motohawk_calibration  nam='Regen_Full'  val=0.7  storage=Calibration  show_more=on  name_source=Use Parameter  data_type=Inherit from 'Default Value'  read_level=1  write_level=1  ovr_cals=on  view_as=Number  enum_struct={'Disabled', 'Enabled'}  vector_style=Wide Row  use_help_units=on  help='Pedal Position where regen is Full (WARNING:CHECK WHAT THE MAX REGEN IS)'  units='%'  use_header_enum=off  row_header_enum={}  col_header_enum={}  use_min_max=on  min_val=0  max_val=1  use_precision=off  precision='1.2'  gain=1  offset=0  exp=1  use_mototune_group=off  mototune_group=motohawk_vardec_path(gcb)
  motohawk_calibration3 : MotoHawk_lib/Calibration & Probing Blocks/motohawk_calibration  nam='Max_Regen_Tq'  val=100  storage=Calibration  show_more=on  name_source=Use Parameter  data_type=Inherit from 'Default Value'  read_level=1  write_level=1  ovr_cals=on  view_as=Number  enum_struct={'Disabled', 'Enabled'}  vector_style=Wide Row  use_help_units=on  help='Max tq regen can apply WARNING: CHECK PEDAL AT MAX TQ'  units='%'  use_header_enum=off  row_header_enum={}  col_header_enum={}  use_min_max=on  min_val=0  max_val=240  use_precision=off  precision='1.2'  gain=1  offset=0  exp=1  use_mototune_group=off  mototune_group=motohawk_vardec_path(gcb)
  motohawk_calibration4 : MotoHawk_lib/Calibration & Probing Blocks/motohawk_calibration  nam='Enable_Regen'  val=0  storage=Calibration  show_more=on  name_source=Use Parameter  data_type=Inherit from 'Default Value'  read_level=1  write_level=1  ovr_cals=on  view_as=Number  enum_struct={'Disabled', 'Enabled'}  vector_style=Wide Row  use_help_units=off  help='Pedal Position where regen is Full'  units='%'  use_header_enum=off  row_header_enum={}  col_header_enum={}  use_min_max=on  min_val=0  max_val=1  use_precision=off  precision='1.2'  gain=1  offset=0  exp=1  use_mototune_group=off  mototune_group=motohawk_vardec_path(gcb)
  motohawk_calibration5 : MotoHawk_lib/Calibration & Probing Blocks/motohawk_calibration  nam='Enable_Coast_Neg_Torque'  val=0  storage=Calibration  show_more=on  name_source=Use Parameter  data_type=Inherit from 'Default Value'  read_level=1  write_level=1  ovr_cals=on  view_as=Number  enum_struct={'Disabled', 'Enabled'}  vector_style=Wide Row  use_help_units=on  help='This allows neg. torque to be applied, depending on vehcild speed, when going from gas to brake'  units=''  use_header_enum=off  row_header_enum={}  col_header_enum={}  use_min_max=on  min_val=0  max_val=1  use_precision=off  precision='1.2'  gain=1  offset=0  exp=1  use_mototune_group=off  mototune_group=motohawk_vardec_path(gcb)
  motohawk_calibration6 : MotoHawk_lib/Calibration & Probing Blocks/motohawk_calibration  nam='Min_Speed_Allow_Coast_NegT'  val=12  storage=Calibration  show_more=on  name_source=Use Parameter  data_type=Inherit from 'Default Value'  read_level=1  write_level=1  ovr_cals=on  view_as=Number  enum_struct={'Disabled', 'Enabled'}  vector_style=Wide Row  use_help_units=on  help='Below this speed, negative torque will not be allowed to cause vehicle drag'  units='MPH'  use_header_enum=off  row_header_enum={}  col_header_enum={}  use_min_max=on  min_val=0  max_val=1  use_precision=off  precision='1.2'  gain=1  offset=0  exp=1  use_mototune_group=off  mototune_group=motohawk_vardec_path(gcb)
  motohawk_calibration7 : MotoHawk_lib/Calibration & Probing Blocks/motohawk_calibration  nam='Max_Coast_Tq'  val=15  storage=Calibration  show_more=on  name_source=Use Parameter  data_type=Inherit from 'Default Value'  read_level=1  write_level=1  ovr_cals=on  view_as=Number  enum_struct={'Disabled', 'Enabled'}  vector_style=Wide Row  use_help_units=on  help='Changing this will change the amount of drag on the vehile when coasting'  units='%'  use_header_enum=off  row_header_enum={}  col_header_enum={}  use_min_max=on  min_val=0  max_val=240  use_precision=off  precision='1.2'  gain=1  offset=0  exp=1  use_mototune_group=off  mototune_group=motohawk_vardec_path(gcb)
  motohawk_calibration8 : MotoHawk_lib/Calibration & Probing Blocks/motohawk_calibration  nam='Max_SOC_For_Coast_Tq_EN'  val=90  storage=Calibration  show_more=on  name_source=Use Parameter  data_type=Inherit from 'Default Value'  read_level=1  write_level=1  ovr_cals=on  view_as=Number  enum_struct={'Disabled', 'Enabled'}  vector_style=Wide Row  use_help_units=on  help='Above this SOC, vehcile will not allow negative torque to be applied when coasting'  units='%'  use_header_enum=off  row_header_enum={}  col_header_enum={}  use_min_max=on  min_val=0  max_val=240  use_precision=off  precision='1.2'  gain=1  offset=0  exp=1  use_mototune_group=off  mototune_group=motohawk_vardec_path(gcb)
  motohawk_override_abs : MotoHawk_lib/Calibration & Probing Blocks/motohawk_override_abs  SystemSampleTime=-1  parent_name='Regen_SOC_Speed_Ramp_ovr'  parent_val=0  show_more=off  name_source=Use Parameter  parent_read_level=1  parent_override_level=1  view_as=Number  enum_struct={'Disabled', 'Enabled'}  use_help_units=off  parent_help=''  parent_units=''  use_min_max=off  parent_min=-inf  parent_max=inf  use_precision=off  parent_precision=''  parent_gain=1  parent_offset=0  parent_exp=1  use_mototune_group=off  parent_group=motohawk_vardec_path(gcb)
  motohawk_probe : MotoHawk_lib/Calibration & Probing Blocks/motohawk_probe  nam='Regen_SOCSpd_Ramp_probe_preOVR'  show_more=off  name_source=Use Parameter  read_level=1  view_as=Number  enum_struct={'Disabled', 'Enabled'}  vector_style=Wide Row  use_help_units=off  help=''  units=''  use_header_enum=off  row_header_enum={}  col_header_enum={}  use_precision=off  precision=''  gain=1  offset=0  exp=1  use_mototune_group=off  mototune_group=motohawk_vardec_path(gcb)
  motohawk_probe1 : MotoHawk_lib/Calibration & Probing Blocks/motohawk_probe  nam='Raw_Regen_Tq_Request'  show_more=off  name_source=Use Parameter  read_level=1  view_as=Number  enum_struct={'Disabled', 'Enabled'}  vector_style=Wide Row  use_help_units=off  help=''  units=''  use_header_enum=off  row_header_enum={}  col_header_enum={}  use_precision=off  precision=''  gain=1  offset=0  exp=1  use_mototune_group=off  mototune_group=motohawk_vardec_path(gcb)
  motohawk_probe2 : MotoHawk_lib/Calibration & Probing Blocks/motohawk_probe  nam='Coast_Down_Tq_Probe'  show_more=off  name_source=Use Parameter  read_level=1  view_as=Number  enum_struct={'Disabled', 'Enabled'}  vector_style=Wide Row  use_help_units=off  help=''  units=''  use_header_enum=off  row_header_enum={}  col_header_enum={}  use_precision=off  precision=''  gain=1  offset=0  exp=1  use_mototune_group=off  mototune_group=motohawk_vardec_path(gcb)
  motohawk_table_2d : MotoHawk_lib/Lookup Tables/motohawk_table_2d  SystemSampleTime=-1  nam='MotoHawkTable2D'  row_nam='StateOfChargePct'  col_nam='MotorSpd'  row_breakpoint_data=[0 85 90 93]  col_breakpoint_data=[0 100 200 400 600 700 800 6800]  table_data=[0 .05 .15 .2 .35 .5 1 1; 0 .05 .15 .2 .35 .5 1 1; 0 .05 .15 .2 .35 .5 .5 .5; 0 0 0 0 0 0 0 0]  show_more=on  row_bp_data_type=Inherit from 'Row Breakpoint Data'  col_bp_data_type=Inherit from 'Column Breakpoint Data'  bp_storage=Constant  table_data_type=Inherit from 'Table Data'  storage=NonAdaptive  read_level=1  write_level=1  ovr_cals=on  use_help=off  help=''  row_bp_units=''  col_bp_units=''  table_units=''  use_min_max=off  row_bp_min_val=-inf  row_bp_max_val=inf  col_bp_min_val=-inf  col_bp_max_val=inf  min_val=-inf  max_val=inf  use_precision=on  use_row_breakpoint=off  rb_precision=''  rb_gain=1  rb_offset=0  rb_exp=1  use_col_breakpoint=off  cb_precision=''  cb_gain=1  cb_offset=0  cb_exp=1  use_table=on  t_precision='1.3'  t_gain=1  t_offset=0  t_exp=1  use_links=off  row_input_name=''  col_input_name=''  output_name=''  use_mototune_group=off  mototune_group=motohawk_vardec_path(gcb)
  RegenTq : Outport
  RegenDisable : Outport  Port=2
  wires:
  Divide/1 -> Saturation2/1
  Gain/1 -> Product/2
  Brake_Pos/1 -> Sum/1
  motohawk_calibration3/1 -> Product/1
  Saturation/1 -> RegenTq/1
  Product/1 -> Product1/2, motohawk_probe1/1
  SOC/1 -> motohawk_table_2d/1, Relational Operator2/1
  RPM/1 -> motohawk_table_2d/2
  motohawk_table_2d/1 -> Saturation1/1
  Saturation1/1 -> motohawk_override_abs/1, motohawk_probe/1
  motohawk_override_abs/1 -> Product1/3
  motohawk_calibration1/1 -> Sum1/1, Sum/2
  Sum/1 -> Divide/1
  motohawk_calibration2/1 -> Sum1/2
  Sum1/1 -> Divide/2
  Saturation2/1 -> Gain/1
  Logical Operator1/1 -> Logical Operator2/1
  motohawk_calibration4/1 -> Logical Operator/1
  RegenDisabled/1 -> Logical Operator1/1, Logical Operator3/1
  Logical Operator/1 -> Logical Operator1/2, Logical Operator3/2
  Logical Operator2/1 -> Product1/1, Product2/1
  motohawk_calibration5/1 -> Product2/2
  Product2/1 -> Relational Operator1/2, motohawk_probe2/1, First Order Low Pass (Tunable)reg/1(in)
  Relational Operator/1 -> Product2/3
  Vehicle Speed/1 -> Relational Operator/1
  motohawk_calibration6/1 -> Relational Operator/2
  motohawk_calibration7/1 -> Gain1/1
  Switch/1 -> Saturation/1
  Product1/1 -> Relational Operator1/1, Switch/1
  Relational Operator2/1 -> Product2/5
  motohawk_calibration8/1 -> Relational Operator2/2
  Relational Operator1/1 -> Switch/2
  Gain1/1 -> Product2/4
  Logical Operator3/1 -> RegenDisable/1
  First Order Low Pass (Tunable)reg/1(out) -> Switch/3
  switch active/1 -> Product2/6
